simulink model "Test_Bit_Multiplexer_4_to_1_NAND"  (R2023a)
settings: Solver=ode45  StartTime=0.0  StopTime=len  RelTol=1e-3  EnableMultiTasking=on
libraries: simulink x2, Bit_Multiplexers_Lib x1
settings Model: Creator=N  LastModifiedBy=Jozko Mrkvicka
settings SolverCC: AlgebraicLoopSolver=TrustRegion
settings DataIOCC: SaveFormat=Array  ReturnWorkspaceOutputs=off
settings OptimizationCC: LifeSpan=inf
settings DebuggingCC: UnconnectedInputMsg=warning  UnconnectedOutputMsg=warning  UnconnectedLineMsg=warning  SFUnexpectedBacktrackingDiag=warning  SFNoUnconditionalDefaultTransitionDiag=warning  SFExecutionAtInitializationDiag=none  ArithmeticOperatorsInVariantConditions=warning
settings HardwareCC: ProdWordSize=32
settings SFSimCC: SimUseLocalCustomCode=off  CustomCodeUndefinedFunction=UseInterfaceOnly
settings RTWCC: RTWUseLocalCustomCode=off
settings CodeAppCC: StateflowObjectComments=on
settings GRTTargetCC: TargetLangStandard=C89/C90 (ANSI)
settings ConfigComp: CovMetricSettings=dw  CovSaveCumulativeToWorkspaceVar=on  CovSaveSingleToWorkspaceVar=on  CovExternalEMLEnable=off

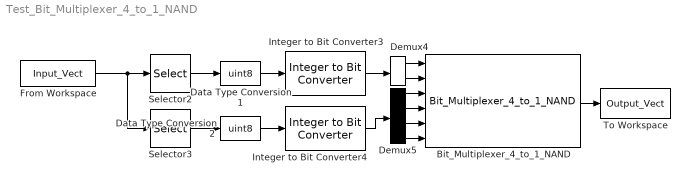
== system Test_Bit_Multiplexer_4_to_1_NAND ==
  Bit_Multiplexer_4_to_1_NAND : Bit_Multiplexers_Lib/Bit_Multiplexers_Lib/Bit_Multiplexer_4_to_1_NAND  SystemSampleTime=-1  VariantActivationTime=update diagram  Latency=0  AutoFrameSizeCalculation=off
  Data Type Conversion1 : DataTypeConversion  OutDataTypeStr=uint8  SaturateOnIntegerOverflow=off  RndMeth=Floor
  Data Type Conversion2 : DataTypeConversion  OutDataTypeStr=uint8  SaturateOnIntegerOverflow=off  RndMeth=Floor
  Demux4 : Demux  Outputs=2
  Demux5 : Demux
  From Workspace : FromWorkspace  VariableName=Input_Vect  SampleTime=1  Interpolate=off  ZeroCross=off  OutputAfterFinalValue=Holding final value
  Integer to Bit Converter3 : simulink/Logic and Bit Operations/Integer to Bit Converter  nbits=2  signedInputValues=Unsigned  bitOrder=MSB first  outDtype=boolean
      settings: LibrarySourceBlock=|
      | commutil2/Integer to Bit
      | Converter
  Integer to Bit Converter4 : simulink/Logic and Bit Operations/Integer to Bit Converter  nbits=4  signedInputValues=Unsigned  bitOrder=MSB first  outDtype=uint8
      settings: LibrarySourceBlock=|
      | commutil2/Integer to Bit
      | Converter
  Selector2 : Selector  IndexMode=Zero-based  InputPortWidth=2  SampleTime=1  IndexOptions=Index vector (dialog)  Indices=0  OutputSizes=1
  Selector3 : Selector  IndexMode=Zero-based  InputPortWidth=2  IndexOptions=Index vector (dialog)  Indices=1  OutputSizes=1
  To Workspace : ToWorkspace  VariableName=Output_Vect  SampleTime=1
  wires:
  Demux4/2 -> Bit_Multiplexer_4_to_1_NAND/2
  Integer to Bit Converter3/1 -> Demux4/1
  Demux5/1 -> Bit_Multiplexer_4_to_1_NAND/3
  Demux5/2 -> Bit_Multiplexer_4_to_1_NAND/4
  Demux5/3 -> Bit_Multiplexer_4_to_1_NAND/5
  Demux5/4 -> Bit_Multiplexer_4_to_1_NAND/6
  Demux4/1 -> Bit_Multiplexer_4_to_1_NAND/1
  From Workspace/1 -> Selector3/1, Selector2/1
  Selector2/1 -> Data Type Conversion1/1
  Selector3/1 -> Data Type Conversion2/1
  Data Type Conversion1/1 -> Integer to Bit Converter3/1
  Data Type Conversion2/1 -> Integer to Bit Converter4/1
  Bit_Multiplexer_4_to_1_NAND/1 -> To Workspace/1
  Integer to Bit Converter4/1 -> Demux5/1
